simulink model "r2_dpa"  (R2012b)
(part 2 of 32)

  gbe3/8(rx_source_ip) -> [gbe_rx_source_ip3]
  gbe3/9(rx_source_port) -> [gbe_rx_source_port3]
  gbe3/12(rx_overrun) -> Terminator25/1
  gbe3/6(rx_data) -> [gbe_rxdata3]
  gbe3/7(rx_valid) -> [gbe_rxvld3]
  gbe3/10(rx_end_of_frame) -> [gbe_rxeof3]
  [gbe_rst] -> gbe2/1(rst)
  [gbe_txd2] -> gbe2/2(tx_data)
  [gbe_txvld2] -> gbe2/3(tx_valid)
  [gbe_txeof2] -> gbe2/6(tx_end_of_frame)
  [gbe_rst] -> gbe3/1(rst)
  [gbe_txd3] -> gbe3/2(tx_data)
  [gbe_txvld3] -> gbe3/3(tx_valid)
  [gbe_txeof3] -> gbe3/6(tx_end_of_frame)
  Constant7/1 -> [gbe_txd2]
  Constant10/1 -> [gbe_txvld2]
  Constant11/1 -> [gbe_txeof2]
  Constant15/1 -> [gbe_txd3]
  Constant12/1 -> [gbe_txvld3]
  Constant14/1 -> [gbe_txeof3]
  [gbe_rxvld2] -> Delay41/1(d)
  [gbe_rxdata2] -> Delay40/1(d)
  [gbe_rxeof2] -> Delay42/1(d)
  Delay40/1(q) -> spead_unpack2/1(pkt_data)
  Delay41/1(q) -> spead_unpack2/2(pkt_valid)
  Delay42/1(q) -> spead_unpack2/3(pkt_eof)
  spead_unpack2/1(pkt_start) -> Terminator34/1
  spead_unpack2/2(data64) -> [spead_data2]
  spead_unpack2/3(valid64) -> [spead_valid2]
  spead_unpack2/4(eof64) -> [spead_eof2]
  spead_unpack2/5(error) -> [spead_error2]
  spead_unpack2/6(hdr_heap_id) -> Terminator29/1
  spead_unpack2/7(hdr_heap_size) -> Terminator30/1
  spead_unpack2/8(hdr_heap_offset) -> Terminator33/1
  spead_unpack2/9(hdr_pkt_len) -> Terminator27/1
  spead_unpack2/11(hdr6_0x4101_DIR) -> [spead_hdr2_2]
  spead_unpack2/12(hdr7_0x4102_DIR) -> [spead_hdr3_2]
  spead_unpack2/13(hdr8_0x4103_DIR) -> [spead_hdr4_2]
  spead_unpack2/14(hdr9_0x4300) -> Terminator37/1
  spead_unpack2/10(hdr5_0x1600_DIR) -> [spead_hdr1_2]
  [gbe_rxvld3] -> Delay44/1(d)
  [gbe_rxdata3] -> Delay43/1(d)
  [gbe_rxeof3] -> Delay45/1(d)
  Delay43/1(q) -> spead_unpack3/1(pkt_data)
  Delay44/1(q) -> spead_unpack3/2(pkt_valid)
  Delay45/1(q) -> spead_unpack3/3(pkt_eof)
  spead_unpack3/1(pkt_start) -> Terminator43/1
  spead_unpack3/2(data64) -> [spead_data3]
  spead_unpack3/3(valid64) -> [spead_valid3]
  spead_unpack3/4(eof64) -> [spead_eof3]
  spead_unpack3/5(error) -> [spead_error3]
  spead_unpack3/6(hdr_heap_id) -> Terminator40/1
  spead_unpack3/7(hdr_heap_size) -> Terminator41/1
  spead_unpack3/8(hdr_heap_offset) -> Terminator42/1
  spead_unpack3/9(hdr_pkt_len) -> Terminator39/1
  spead_unpack3/11(hdr6_0x4101_DIR) -> [spead_hdr2_3]
  spead_unpack3/12(hdr7_0x4102_DIR) -> [spead_hdr3_3]
  spead_unpack3/13(hdr8_0x4103_DIR) -> [spead_hdr4_3]
  spead_unpack3/14(hdr9_0x4300) -> Terminator44/1
  spead_unpack3/10(hdr5_0x1600_DIR) -> [spead_hdr1_3]
  [cnt_rst] -> Subsystem1/1(rst)
  [spead_error2] -> Subsystem1/4(flag)
  [spead_eof2] -> Subsystem1/3(eof)
  [spead_valid2] -> Subsystem1/2(we)
  Subsystem1/1(rx_cnt) -> rx_cnt2/1(out_reg)
  Subsystem1/2(err_cnt) -> rx_err_cnt2/1(out_reg)
  Subsystem1/3(desterr_cnt) -> dest_err_cnt2/1(out_reg)
  [pre_rx_dest_err2] -> Subsystem1/5(dest_err)
  [cnt_rst] -> Subsystem3/1(rst)
  [spead_error3] -> Subsystem3/4(flag)
  [spead_eof3] -> Subsystem3/3(eof)
  [spead_valid3] -> Subsystem3/2(we)
  Subsystem3/1(rx_cnt) -> rx_cnt3/1(out_reg)
  Subsystem3/2(err_cnt) -> rx_err_cnt3/1(out_reg)
  Subsystem3/3(desterr_cnt) -> dest_err_cnt3/1(out_reg)
  [pre_rx_dest_err3] -> Subsystem3/5(dest_err)
  Constant18/1 -> gbe3/4(tx_dest_ip)
  Constant19/1 -> gbe3/5(tx_dest_port)
  Constant16/1 -> gbe2/4(tx_dest_ip)
  Constant17/1 -> gbe2/5(tx_dest_port)
  vacctvg_control/1(in_sync_sel) -> pipeline65/1(d)
  vacctvg_control/2(in_valid_sel) -> pipeline62/1(d)
  vacctvg_control/3(in_data_sel) -> pipeline66/1(d)
  vacctvg_control/4(in_reset) -> pipeline64/1(d)
  vacctvg_control/5(in_ctr_en) -> pipeline69/1(d)
  vacctvg_control/6(in_vector_en) -> pipeline67/1(d)
  vacctvg_control/7(in_pulse_en) -> pipeline70/1(d)
  pipeline65/1(q) -> [vacctvg_sync_sel]
  pipeline62/1(q) -> [vacctvg_valid_sel]
  pipeline64/1(q) -> [vacctvg_reset]
  pipeline66/1(q) -> [vacctvg_data_sel]
  pipeline67/1(q) -> [vacctvg_vector_en]
  pipeline69/1(q) -> [vacctvg_ctr_en]
  pipeline70/1(q) -> [vacctvg_pulse_en]
  pipeline68/1(q) -> [vacctvg_vbs_rst0]
  vacctvg_control/8(in_vbs_rst0) -> pipeline68/1(d)
  pipeline71/1(q) -> [vacctvg_vbs_rst1]
  pipeline63/1(q) -> [vacctvg_vbs_rst2]
  pipeline72/1(q) -> [vacctvg_vbs_rst3]
  vacctvg_control/9(in_vbs_rst1) -> pipeline71/1(d)
  vacctvg_control/10(in_vbs_rst2) -> pipeline63/1(d)
  vacctvg_control/11(in_vbs_rst3) -> pipeline72/1(d)
  Constant23/1 -> [gbe_txvld0]
  Constant24/1 -> [gbe_txstart0]
  Constant25/1 -> [gbe_txeof0]
  Constant1/1 -> [gbe_txd0]
  Constant26/1 -> [gbe_txport0]
  Constant27/1 -> [gbe_txip0]
  Constant28/1 -> [gbe_ipsel0]
  Constant29/1 -> [gbe_txip1]
  Constant30/1 -> [gbe_txport1]
  Constant31/1 -> [gbe_txd1]
  Constant32/1 -> [gbe_txvld1]
  Constant33/1 -> [gbe_txeof1]
  [gbe_rxdata1] -> pipeline27/1(d)
  gbe1/8(rx_source_ip) -> [gbe_rx_source_ip1]
  gbe1/9(rx_source_port) -> [gbe_rx_source_port1]
  [gbe_rxdata2] -> pipeline34/1(d)
  [gbe_rx_source_ip2] -> pipeline35/1(d)
  [gbe_rx_source_port2] -> pipeline36/1(d)
  [gbe_rxvld2] -> pipeline38/1(d), pipeline39/1(d)
  gbe2/8(rx_source_ip) -> [gbe_rx_source_ip2]
  gbe2/9(rx_source_port) -> [gbe_rx_source_port2]
  [gbe_rx_source_ip3] -> pipeline42/1(d)
  spead_unpack0/15(error_debug) -> [spead_error_db0]
  spead_unpack1/15(error_debug) -> [spead_error_db1]
  spead_unpack2/15(error1) -> [spead_error_db2]
  spead_unpack3/15(error_debug) -> [spead_error_db3]
  [spead_error_db2] -> pipeline37/1(d)
  [gbe_rxdata3] -> pipeline41/1(d)
  [gbe_rx_source_port3] -> pipeline43/1(d)
  [gbe_rxvld3] -> pipeline46/1(d), pipeline45/1(d)
  [spead_error_db3] -> pipeline44/1(d)
  [gbe_rxvld1] -> pipeline32/1(d), pipeline31/1(d)
  [gbe_rx_source_ip1] -> pipeline28/1(d)
  [gbe_rx_source_port1] -> pipeline29/1(d)
  [spead_error_db1] -> pipeline30/1(d)
  [gbe_rxdata0] -> pipeline26/1(d)
  [gbe_rx_source_ip0] -> pipeline24/1(d)
  [gbe_rx_source_port0] -> pipeline23/1(d)
  [gbe_rxvld0] -> pipeline9/1(d), pipeline10/1(d)
  [spead_error_db0] -> pipeline14/1(d)
  pipeline/1(q) -> ss_gbe4/7(stop)
  pipeline9/1(q) -> ss_gbe4/6(trig)
  pipeline10/1(q) -> ss_gbe4/5(we)
  pipeline14/1(q) -> ss_gbe4/4(in_debug)
  pipeline23/1(q) -> ss_gbe4/3(in_src_port)
  pipeline24/1(q) -> ss_gbe4/2(in_src_ip)
  pipeline26/1(q) -> ss_gbe4/1(in_data64)
  pipeline27/1(q) -> ss_gbe1/1(in_data64)
  pipeline28/1(q) -> ss_gbe1/2(in_src_ip)
  pipeline29/1(q) -> ss_gbe1/3(in_src_port)
  pipeline30/1(q) -> ss_gbe1/4(in_debug)
  pipeline31/1(q) -> ss_gbe1/5(we)
  pipeline32/1(q) -> ss_gbe1/6(trig)
  pipeline33/1(q) -> ss_gbe1/7(stop)
  pipeline34/1(q) -> ss_gbe2/1(in_data64)
  pipeline35/1(q) -> ss_gbe2/2(in_src_ip)
  pipeline36/1(q) -> ss_gbe2/3(in_src_port)
  pipeline37/1(q) -> ss_gbe2/4(in_debug)
  pipeline38/1(q) -> ss_gbe2/5(we)
  pipeline39/1(q) -> ss_gbe2/6(trig)
  pipeline40/1(q) -> ss_gbe2/7(stop)
  pipeline41/1(q) -> ss_gbe3/1(in_data64)
  pipeline42/1(q) -> ss_gbe3/2(in_src_ip)
  pipeline43/1(q) -> ss_gbe3/3(in_src_port)
  pipeline44/1(q) -> ss_gbe3/4(in_debug)
  pipeline45/1(q) -> ss_gbe3/5(we)
  pipeline46/1(q) -> ss_gbe3/6(trig)
  pipeline47/1(q) -> ss_gbe3/7(stop)
  Logical/1 -> pipeline33/1(d)
  [spead_error1] -> Logical/1
  [ss_man_stop] -> Logical/2
  Logical1/1 -> pipeline40/1(d)
  [spead_error2] -> Logical1/1
  [ss_man_stop] -> Logical1/2
  [spead_error0] -> Logical2/1
  [ss_man_stop] -> Logical2/2
  Logical2/1 -> pipeline/1(d)
  [spead_error3] -> Logical3/1
  [ss_man_stop] -> Logical3/2
  Logical3/1 -> pipeline47/1(d)
  ss_man_stop/1(in_reg) -> Delay1/1(d)
  Delay1/1(q) -> [ss_man_stop]
